simulink model "NPC_inverter_TS_203864"  (R2023b)
settings: Solver=ode4  StartTime=0.0  StopTime=Tsim  FixedStep=Ts  RelTol=1e-3
InitFcn:
  | run('param.m');
values from neighbouring files (symbols this model uses):
  f = 50    [param_nfE.m]
  mmax = 1    [param_nfE.m]
  mmin = -1    [param_nfE.m]
  TA = Tc    (= 0.000125)    [param_nfE.m]
  Tc = 1/fc    (= 0.000125)    [param_nfE.m]
  Umax = Ud/2    (= 350)    [param_nfE.m]
undefined symbols (not defined in the file or in its folder): plecs
libraries: simulink x12, plecslib x5
settings Model: Creator=timsp  LastModifiedBy=timsp

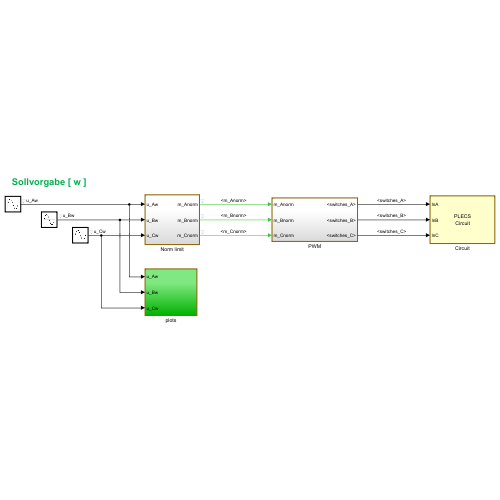
[thumbnail: Simulink's stored preview of the top-level diagram]
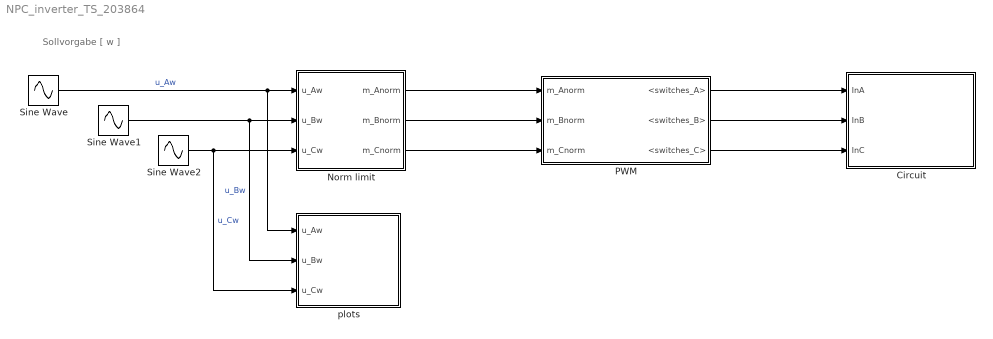
== system NPC_inverter_TS_203864 ==
  note: Sollvorgabe [ w ]
  Circuit : Subsystem  LoadFcn=plecs('sl', 200);  InitFcn=plecs('sl', 214);  StartFcn=plecs('sl', 208);  StopFcn=plecs('sl', 209);  mask(PlecsCircuit){PLECSData=<binary blob, 5248 chars, not shown>}
      mask prompts: PLECSData "PLECS Data (Do not delete or modify!)"
      mask init:
      | % PLACE CUSTOM INITIALIZATIONS ABOVE
      | % DO NOT REMOVE
      | plecs('sl', 215);
      | % DO NOT REMOVE
      settings: CopyFcn=plecs('sl', 203);  DeleteFcn=plecs('sl', 205);  UndoDeleteFcn=plecs('sl', 206);  PreSaveFcn=plecs('sl', 211);  PostSaveFcn=plecs('sl', 201);  NameChangeFcn=plecs('sl', 210);  DestroyFcn=plecs('sl', 207);  PreCopyFcn=plecs('sl', 216);  OpenFcn=plecs('sl', 202);  ErrorFcn=plerrorfcn
      mask Help: eval('plecs(''help'', ''qthelp:///creatingacircuit.html'')')
      mask Display: disp('PLECS\nCircuit')
  Norm limit : Subsystem
  PWM : Subsystem
  Sine Wave : Sin  Amplitude=Umax  Frequency=2*pi*f  Phase=pi/2  SampleTime=0
  Sine Wave1 : Sin  Amplitude=Umax  Frequency=2*pi*f  Phase=-2*pi/3+pi/2  SampleTime=0
  Sine Wave2 : Sin  Amplitude=Umax  Frequency=2*pi*f  Phase=-4*pi/3+pi/2  SampleTime=0
  plots : Subsystem
  wires:
  PWM/1(<switches_A>) -> Circuit/1(InA)
  PWM/2(<switches_B>) -> Circuit/2(InB)
  PWM/3(<switches_C>) -> Circuit/3(InC)
  Norm limit/1(m_Anorm) -> PWM/1(m_Anorm)
  Norm limit/2(m_Bnorm) -> PWM/2(m_Bnorm)
  Norm limit/3(m_Cnorm) -> PWM/3(m_Cnorm)
  Sine Wave/1 -> plots/1(u_Aw), Norm limit/1(u_Aw)  "u_Aw"
  Sine Wave1/1 -> plots/2(u_Bw), Norm limit/2(u_Bw)  "u_Bw"
  Sine Wave2/1 -> plots/3(u_Cw), Norm limit/3(u_Cw)  "u_Cw"

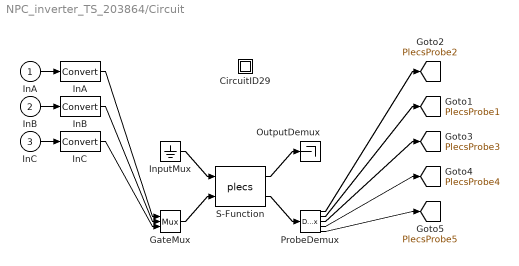
== system NPC_inverter_TS_203864/Circuit ==
  InA : Inport  PortDimensions=4
  InB : Inport  Port=2  PortDimensions=4
  InC : Inport  Port=3  PortDimensions=4
  " CircuitID29 " : Subsystem
  " GateMux " : Mux  Inputs=[ 4 4 4 ]
  " InA " : DataTypeConversion
  " InB " : DataTypeConversion
  " InC " : DataTypeConversion
  " InputMux " : Ground
  " OutputDemux " : Terminator
  " ProbeDemux " : Demux  Outputs=[ 3 3 3 1 3 ]
  " S-Function " : S-Function  FunctionName=plecs  SFunctionDeploymentMode=off  EnableBusSupport=off
  tag scope: PlecsProbe1=global, PlecsProbe2=global, PlecsProbe3=global, PlecsProbe4=global, PlecsProbe5=global
  wires:
  " InputMux "/1 -> " S-Function "/1
  " GateMux "/1 -> " S-Function "/2
  " S-Function "/1 -> " OutputDemux "/1
  " S-Function "/2 -> " ProbeDemux "/1
  InA/1 -> " InA "/1
  " InA "/1 -> " GateMux "/1
  InB/1 -> " InB "/1
  " InB "/1 -> " GateMux "/2
  InC/1 -> " InC "/1
  " InC "/1 -> " GateMux "/3
  " ProbeDemux "/1 -> [PlecsProbe2]
  " ProbeDemux "/2 -> [PlecsProbe1]
  " ProbeDemux "/3 -> [PlecsProbe3]
  " ProbeDemux "/4 -> [PlecsProbe4]
  " ProbeDemux "/5 -> [PlecsProbe5]

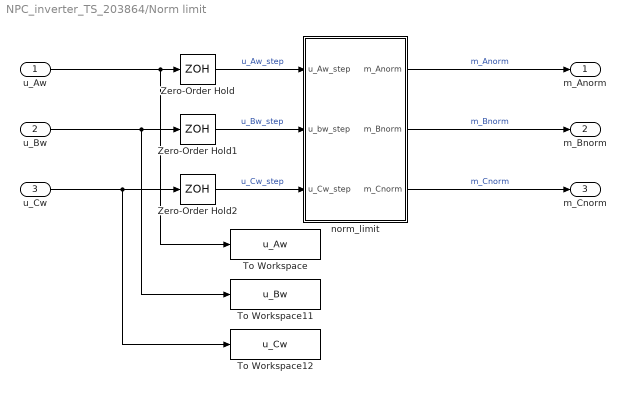
== system NPC_inverter_TS_203864/Norm limit ==
  u_Aw : Inport
  u_Bw : Inport  Port=2
  u_Cw : Inport  Port=3
  To Workspace : ToWorkspace  VariableName=u_Aw  SampleTime=-1
      settings: Save2DSignal=2-D array (concatenate along first dimension)
  To Workspace11 : ToWorkspace  VariableName=u_Bw  SampleTime=-1
      settings: Save2DSignal=2-D array (concatenate along first dimension)
  To Workspace12 : ToWorkspace  VariableName=u_Cw  SampleTime=-1
      settings: Save2DSignal=2-D array (concatenate along first dimension)
  Zero-Order Hold : ZeroOrderHold  SampleTime=TA
  Zero-Order Hold1 : ZeroOrderHold  SampleTime=TA
  Zero-Order Hold2 : ZeroOrderHold  SampleTime=TA
  norm_limit : Subsystem
  m_Anorm : Outport
  m_Bnorm : Outport  Port=2
  m_Cnorm : Outport  Port=3
  wires:
  u_Cw/1 -> To Workspace12/1, Zero-Order Hold2/1
  u_Bw/1 -> To Workspace11/1, Zero-Order Hold1/1
  norm_limit/3(m_Cnorm) -> m_Cnorm/1  "m_Cnorm"
  Zero-Order Hold1/1 -> norm_limit/2(u_bw_step)  "u_Bw_step"
  norm_limit/2(m_Bnorm) -> m_Bnorm/1  "m_Bnorm"
  Zero-Order Hold/1 -> norm_limit/1(u_Aw_step)  "u_Aw_step"
  Zero-Order Hold2/1 -> norm_limit/3(u_Cw_step)  "u_Cw_step"
  norm_limit/1(m_Anorm) -> m_Anorm/1  "m_Anorm"
  u_Aw/1 -> To Workspace/1, Zero-Order Hold/1

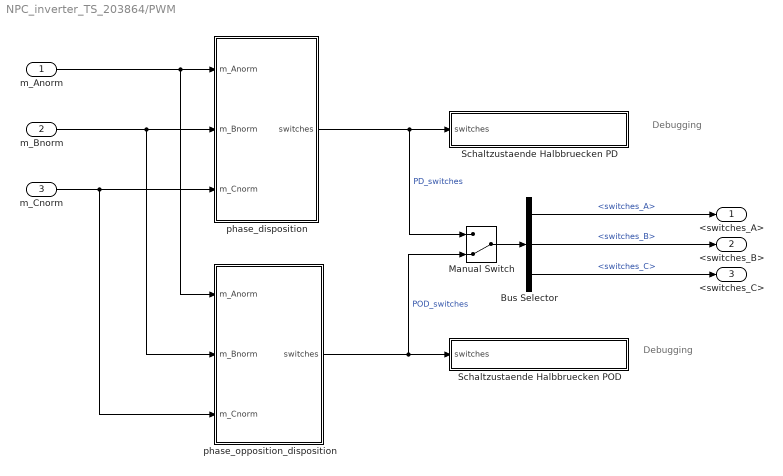
== system NPC_inverter_TS_203864/PWM ==
  note: Debugging
  note: Debugging
  m_Anorm : Inport
  m_Bnorm : Inport  Port=2
  m_Cnorm : Inport  Port=3
  Bus Selector : BusSelector  OutputSignals=switches_A,switches_B,switches_C
  Manual Switch : ManualSwitch  CurrentSetting=0
  Schaltzustaende Halbbruecken PD : Subsystem
  Schaltzustaende Halbbruecken POD : Subsystem
  phase_disposition : Subsystem  TreatAsAtomicUnit=on
  phase_opposition_disposition : Subsystem  TreatAsAtomicUnit=on
  <switches_A> : Outport
  <switches_B> : Outport  Port=2
  <switches_C> : Outport  Port=3
  wires:
  m_Bnorm/1 -> phase_disposition/2(m_Bnorm), phase_opposition_disposition/2(m_Bnorm)
  phase_disposition/1(switches) -> Schaltzustaende Halbbruecken PD/1(switches), Manual Switch/1  "PD_switches"
  phase_opposition_disposition/1(switches) -> Manual Switch/2, Schaltzustaende Halbbruecken POD/1(switches)  "POD_switches"
  Bus Selector/3 -> <switches_C>/1  "<switches_C>"
  m_Cnorm/1 -> phase_opposition_disposition/3(m_Cnorm), phase_disposition/3(m_Cnorm)
  m_Anorm/1 -> phase_opposition_disposition/1(m_Anorm), phase_disposition/1(m_Anorm)
  Bus Selector/1 -> <switches_A>/1  "<switches_A>"
  Manual Switch/1 -> Bus Selector/1
  Bus Selector/2 -> <switches_B>/1  "<switches_B>"

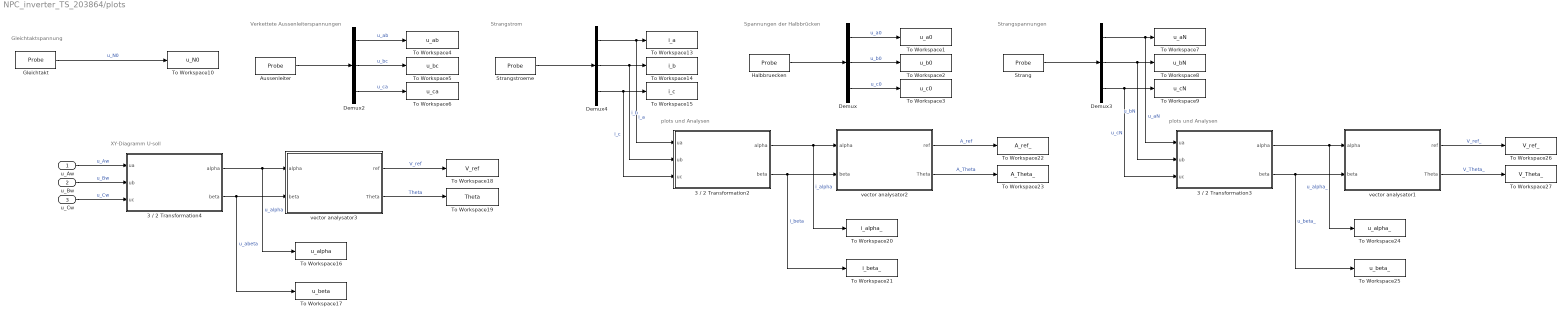
== system NPC_inverter_TS_203864/plots ==
  note: Gleichtaktspannung
  note: Spannungen der Halbbrücken
  note: Verkettete Aussenleiterspannungen
  note: Strangspannungen
  note: Strangstrom
  note: plots und Analysen
  note: plots und Analysen
  note: XY-Diagramm U-soll
  u_Aw : Inport
  u_Bw : Inport  Port=2
  u_Cw : Inport  Port=3
  3 / 2 Transformation2 : MATLAB Function  TreatAsAtomicUnit=on
  3 / 2 Transformation3 : MATLAB Function  TreatAsAtomicUnit=on
  3 / 2 Transformation4 : MATLAB Function  TreatAsAtomicUnit=on
  Aussenleiter : plecslib/Probe  tagno=1
      settings: SourceProductName=PLECS
  Demux{,2..4} (4 alike) : Demux  Outputs=3
  Gleichtakt : plecslib/Probe  tagno=4
      settings: SourceProductName=PLECS
  Halbbruecken : plecslib/Probe  tagno=2
      settings: SourceProductName=PLECS
  Strang : plecslib/Probe  tagno=3
      settings: SourceProductName=PLECS
  Strangstroeme : plecslib/Probe  tagno=5
      settings: SourceProductName=PLECS
  To Workspace1 : ToWorkspace  VariableName=u_a0  SampleTime=-1
  To Workspace10 : ToWorkspace  VariableName=u_N0  SampleTime=-1
  To Workspace13 : ToWorkspace  VariableName=i_a  SampleTime=-1
  To Workspace14 : ToWorkspace  VariableName=i_b  SampleTime=-1
  To Workspace15 : ToWorkspace  VariableName=i_c  SampleTime=-1
  To Workspace16 : ToWorkspace  VariableName=u_alpha  SampleTime=-1
  To Workspace17 : ToWorkspace  VariableName=u_beta  SampleTime=-1
  To Workspace18 : ToWorkspace  VariableName=V_ref  SampleTime=-1
  To Workspace19 : ToWorkspace  VariableName=Theta  SampleTime=-1
  To Workspace2 : ToWorkspace  VariableName=u_b0  SampleTime=-1
  To Workspace20 : ToWorkspace  VariableName=i_alpha_  SampleTime=-1
  To Workspace21 : ToWorkspace  VariableName=i_beta_  SampleTime=-1
  To Workspace22 : ToWorkspace  VariableName=A_ref_  SampleTime=-1
  To Workspace23 : ToWorkspace  VariableName=A_Theta_  SampleTime=-1
  To Workspace24 : ToWorkspace  VariableName=u_alpha_  SampleTime=-1
  To Workspace25 : ToWorkspace  VariableName=u_beta_  SampleTime=-1
  To Workspace26 : ToWorkspace  VariableName=V_ref_  SampleTime=-1
  To Workspace27 : ToWorkspace  VariableName=V_Theta_  SampleTime=-1
  To Workspace3 : ToWorkspace  VariableName=u_c0  SampleTime=-1
  To Workspace4 : ToWorkspace  VariableName=u_ab  SampleTime=-1
  To Workspace5 : ToWorkspace  VariableName=u_bc  SampleTime=-1
  To Workspace6 : ToWorkspace  VariableName=u_ca  SampleTime=-1
  To Workspace7 : ToWorkspace  VariableName=u_aN  SampleTime=-1
  To Workspace8 : ToWorkspace  VariableName=u_bN  SampleTime=-1
  To Workspace9 : ToWorkspace  VariableName=u_cN  SampleTime=-1
  vector analysator1 : MATLAB Function  TreatAsAtomicUnit=on
  vector analysator2 : MATLAB Function  TreatAsAtomicUnit=on
  vector analysator3 : MATLAB Function  TreatAsAtomicUnit=on
  wires:
  Demux3/3 -> 3 / 2 Transformation3/3(uc), To Workspace9/1  "u_cN"
  Demux2/1 -> To Workspace4/1  "u_ab"
  Demux2/2 -> To Workspace5/1  "u_bc"
  Aussenleiter/1 -> Demux2/1
  vector analysator1/2(Theta) -> To Workspace27/1  "V_Theta_"
  Demux4/2 -> 3 / 2 Transformation2/2(ub), To Workspace14/1  "i_b"
  Demux3/2 -> 3 / 2 Transformation3/2(ub), To Workspace8/1  "u_bN"
  3 / 2 Transformation3/2(beta) -> vector analysator1/2(beta), To Workspace25/1  "u_beta_"
  Strangstroeme/1 -> Demux4/1
  Demux/1 -> To Workspace1/1  "u_a0"
  Gleichtakt/1 -> To Workspace10/1  "u_N0"
  Demux/2 -> To Workspace2/1  "u_b0"
  Demux4/3 -> 3 / 2 Transformation2/3(uc), To Workspace15/1  "i_c"
  Demux2/3 -> To Workspace6/1  "u_ca"
  3 / 2 Transformation3/1(alpha) -> vector analysator1/1(alpha), To Workspace24/1  "u_alpha_"
  3 / 2 Transformation2/2(beta) -> vector analysator2/2(beta), To Workspace21/1  "i_beta"
  vector analysator2/2(Theta) -> To Workspace23/1  "A_Theta"
  Demux4/1 -> 3 / 2 Transformation2/1(ua), To Workspace13/1  "i_a"
  vector analysator2/1(ref) -> To Workspace22/1  "A_ref"
  3 / 2 Transformation2/1(alpha) -> vector analysator2/1(alpha), To Workspace20/1  "i_alpha"
  vector analysator1/1(ref) -> To Workspace26/1  "V_ref_"
  Strang/1 -> Demux3/1
  Demux3/1 -> 3 / 2 Transformation3/1(ua), To Workspace7/1  "u_aN"
  Halbbruecken/1 -> Demux/1
  Demux/3 -> To Workspace3/1  "u_c0"
  vector analysator3/2(Theta) -> To Workspace19/1  "Theta"
  u_Cw/1 -> 3 / 2 Transformation4/3(uc)  "u_Cw"
  3 / 2 Transformation4/2(beta) -> vector analysator3/2(beta), To Workspace17/1  "u_abeta"
  vector analysator3/1(ref) -> To Workspace18/1  "V_ref"
  3 / 2 Transformation4/1(alpha) -> vector analysator3/1(alpha), To Workspace16/1  "u_alpha"
  u_Bw/1 -> 3 / 2 Transformation4/2(ub)  "u_Bw"
  u_Aw/1 -> 3 / 2 Transformation4/1(ua)  "u_Aw"

== system NPC_inverter_TS_203864/Circuit/ CircuitID29  ==

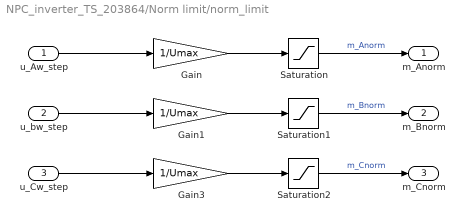
== system NPC_inverter_TS_203864/Norm limit/norm_limit ==
  u_Aw_step : Inport
  u_bw_step : Inport  Port=2
  u_Cw_step : Inport  Port=3
  Gain : Gain  Gain=1/Umax
  Gain1 : Gain  Gain=1/Umax
  Gain3 : Gain  Gain=1/Umax
  Saturation : Saturate  UpperLimit=mmax  LowerLimit=mmin
  Saturation1 : Saturate  UpperLimit=mmax  LowerLimit=mmin
  Saturation2 : Saturate  UpperLimit=mmax  LowerLimit=mmin
  m_Anorm : Outport
  m_Bnorm : Outport  Port=2
  m_Cnorm : Outport  Port=3
  wires:
  Gain/1 -> Saturation/1
  Gain3/1 -> Saturation2/1
  u_Cw_step/1 -> Gain3/1
  Gain1/1 -> Saturation1/1
  u_bw_step/1 -> Gain1/1
  u_Aw_step/1 -> Gain/1
  Saturation/1 -> m_Anorm/1  "m_Anorm"
  Saturation1/1 -> m_Bnorm/1  "m_Bnorm"
  Saturation2/1 -> m_Cnorm/1  "m_Cnorm"

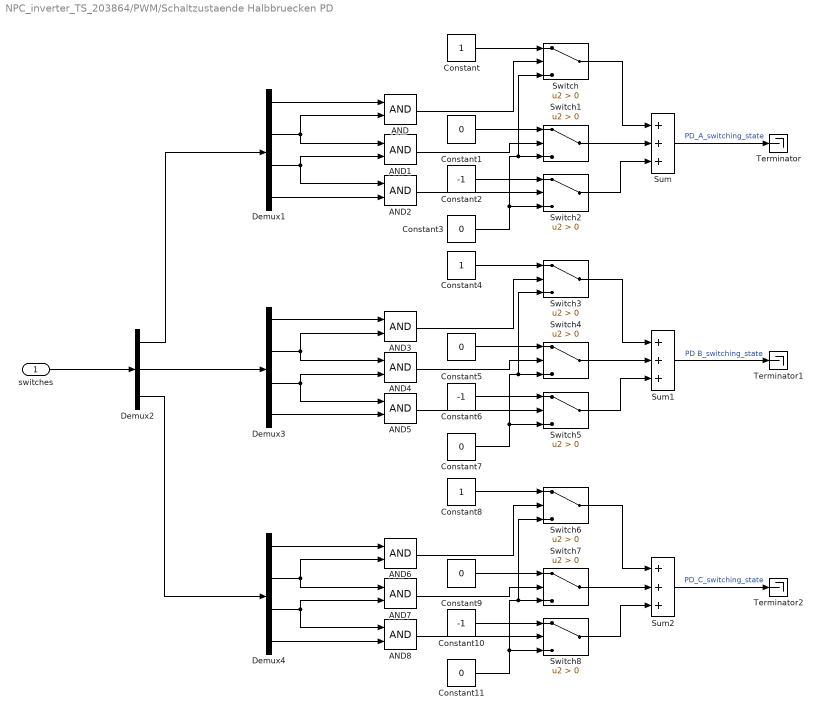
== system NPC_inverter_TS_203864/PWM/Schaltzustaende Halbbruecken PD ==
  switches : Inport
  AND{,1..8} (9 alike) : Logic  AllPortsSameDT=off  OutDataTypeStr=boolean
  Constant : Constant
  Constant{1,3,5,7,9,11} (6 alike) : Constant  Value=0
  Constant10 : Constant  Value=-1
  Constant2 : Constant  Value=-1
  Constant4 : Constant
  Constant6 : Constant  Value=-1
  Constant8 : Constant
  Demux1 : Demux
  Demux2 : Demux  Outputs=3
  Demux3 : Demux
  Demux4 : Demux
  Sum : Sum  Inputs=+++
  Sum1 : Sum  Inputs=+++
  Sum2 : Sum  Inputs=+++
  Switch{,1..8} (9 alike) : Switch  Criteria=u2 > Threshold  SaturateOnIntegerOverflow=off  InputSameDT=off
  Terminator : Terminator
  Terminator1 : Terminator
  Terminator2 : Terminator
  wires:
  Sum2/1 -> Terminator2/1  "PD_C_switching_state"
  Switch8/1 -> Sum2/3
  Switch7/1 -> Sum2/2
  Switch6/1 -> Sum2/1
  Constant11/1 -> Switch8/3, Switch7/3, Switch6/3
  Constant10/1 -> Switch8/1
  AND8/1 -> Switch8/2
  Constant9/1 -> Switch7/1
  AND7/1 -> Switch7/2
  Constant8/1 -> Switch6/1
  AND6/1 -> Switch6/2
  Demux4/4 -> AND8/2
  Demux4/3 -> AND7/2, AND8/1
  Demux4/2 -> AND6/2, AND7/1
  Demux4/1 -> AND6/1
  Demux3/1 -> AND3/1
  Demux3/2 -> AND4/1, AND3/2
  Demux3/3 -> AND5/1, AND4/2
  Demux3/4 -> AND5/2
  AND3/1 -> Switch3/2
  Constant4/1 -> Switch3/1
  AND4/1 -> Switch4/2
  Constant5/1 -> Switch4/1
  AND5/1 -> Switch5/2
  Constant6/1 -> Switch5/1
  Constant7/1 -> Switch3/3, Switch4/3, Switch5/3
  Switch3/1 -> Sum1/1
  Switch4/1 -> Sum1/2
  Switch5/1 -> Sum1/3
  Sum1/1 -> Terminator1/1  "PD B_switching_state"
  Sum/1 -> Terminator/1  "PD_A_switching_state"
  Switch2/1 -> Sum/3
  Switch1/1 -> Sum/2
  Switch/1 -> Sum/1
  Constant3/1 -> Switch2/3, Switch1/3, Switch/3
  Constant2/1 -> Switch2/1
  AND2/1 -> Switch2/2
  Constant1/1 -> Switch1/1
  AND1/1 -> Switch1/2
  Constant/1 -> Switch/1
  AND/1 -> Switch/2
  Demux2/2 -> Demux3/1
  Demux1/4 -> AND2/2
  Demux1/3 -> AND1/2, AND2/1
  Demux1/2 -> AND/2, AND1/1
  Demux1/1 -> AND/1
  Demux2/3 -> Demux4/1
  Demux2/1 -> Demux1/1
  switches/1 -> Demux2/1

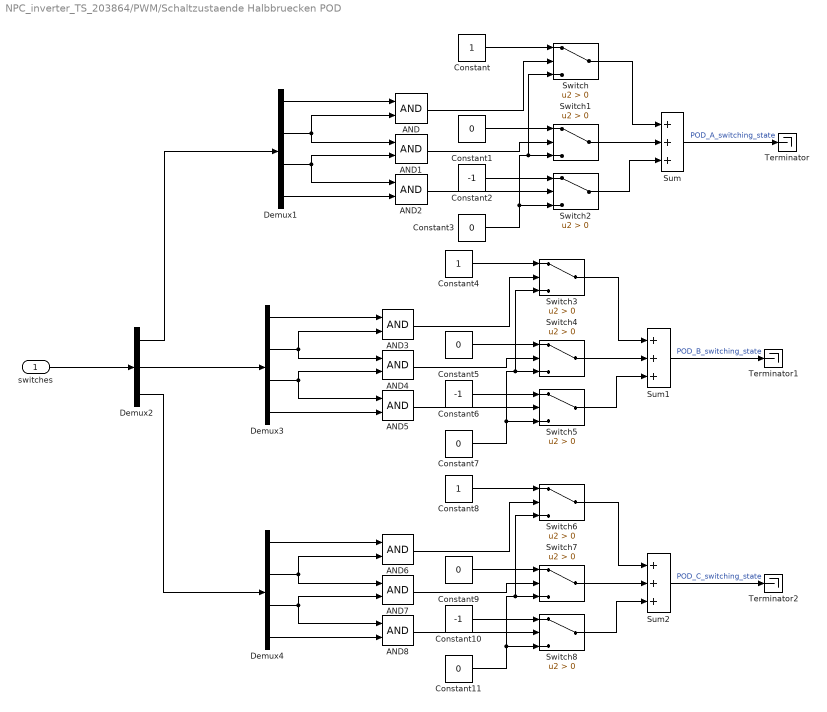
== system NPC_inverter_TS_203864/PWM/Schaltzustaende Halbbruecken POD ==
  switches : Inport
  AND{,1..8} (9 alike) : Logic  AllPortsSameDT=off  OutDataTypeStr=boolean
  Constant : Constant
  Constant{1,3,5,7,9,11} (6 alike) : Constant  Value=0
  Constant10 : Constant  Value=-1
  Constant2 : Constant  Value=-1
  Constant4 : Constant
  Constant6 : Constant  Value=-1
  Constant8 : Constant
  Demux1 : Demux
  Demux2 : Demux  Outputs=3
  Demux3 : Demux
  Demux4 : Demux
  Sum : Sum  Inputs=+++
  Sum1 : Sum  Inputs=+++
  Sum2 : Sum  Inputs=+++
  Switch{,1..8} (9 alike) : Switch  Criteria=u2 > Threshold  SaturateOnIntegerOverflow=off  InputSameDT=off
  Terminator : Terminator
  Terminator1 : Terminator
  Terminator2 : Terminator
  wires:
  switches/1 -> Demux2/1
  Demux2/1 -> Demux1/1
  Demux2/3 -> Demux4/1
  Demux1/1 -> AND/1
  Demux1/2 -> AND1/1, AND/2
  Demux1/3 -> AND2/1, AND1/2
  Demux1/4 -> AND2/2
  Demux2/2 -> Demux3/1
  AND/1 -> Switch/2
  Constant/1 -> Switch/1
  AND1/1 -> Switch1/2
  Constant1/1 -> Switch1/1
  AND2/1 -> Switch2/2
  Constant2/1 -> Switch2/1
  Constant3/1 -> Switch/3, Switch1/3, Switch2/3
  Switch/1 -> Sum/1
  Switch1/1 -> Sum/2
  Switch2/1 -> Sum/3
  Sum/1 -> Terminator/1  "POD_A_switching_state"
  Sum1/1 -> Terminator1/1  "POD_B_switching_state"
  Switch5/1 -> Sum1/3
  Switch4/1 -> Sum1/2
  Switch3/1 -> Sum1/1
  Constant7/1 -> Switch5/3, Switch4/3, Switch3/3
  Constant6/1 -> Switch5/1
  AND5/1 -> Switch5/2
  Constant5/1 -> Switch4/1
  AND4/1 -> Switch4/2
  Constant4/1 -> Switch3/1
  AND3/1 -> Switch3/2
  Demux3/4 -> AND5/2
  Demux3/3 -> AND4/2, AND5/1
  Demux3/2 -> AND3/2, AND4/1
  Demux3/1 -> AND3/1
  Demux4/1 -> AND6/1
  Demux4/2 -> AND7/1, AND6/2
  Demux4/3 -> AND8/1, AND7/2
  Demux4/4 -> AND8/2
  AND6/1 -> Switch6/2
  Constant8/1 -> Switch6/1
  AND7/1 -> Switch7/2
  Constant9/1 -> Switch7/1
  AND8/1 -> Switch8/2
  Constant10/1 -> Switch8/1
  Constant11/1 -> Switch6/3, Switch7/3, Switch8/3
  Switch6/1 -> Sum2/1
  Switch7/1 -> Sum2/2
  Switch8/1 -> Sum2/3
  Sum2/1 -> Terminator2/1  "POD_C_switching_state"

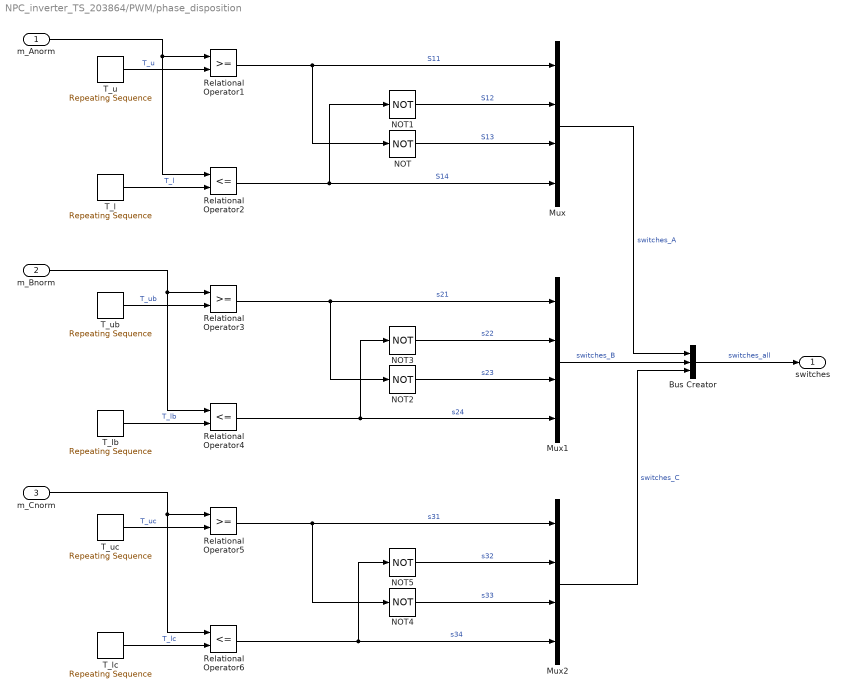
== system NPC_inverter_TS_203864/PWM/phase_disposition ==
  m_Anorm : Inport
  m_Bnorm : Inport  Port=2
  m_Cnorm : Inport  Port=3
  Bus Creator : BusCreator  Inputs=3
  Mux : Mux
  Mux1 : Mux
  Mux2 : Mux
  NOT{,1..5} (6 alike) : Logic  Operator=NOT  AllPortsSameDT=off  OutDataTypeStr=boolean
  Relational Operator1 : RelationalOperator  OutDataTypeStr=boolean  RndMeth=Simplest  InputSameDT=off
  Relational Operator2 : RelationalOperator  Operator=<=  OutDataTypeStr=boolean  RndMeth=Simplest  InputSameDT=off
  Relational Operator3 : RelationalOperator  OutDataTypeStr=boolean  RndMeth=Simplest  InputSameDT=off
  Relational Operator4 : RelationalOperator  Operator=<=  OutDataTypeStr=boolean  RndMeth=Simplest  InputSameDT=off
  Relational Operator5 : RelationalOperator  OutDataTypeStr=boolean  RndMeth=Simplest  InputSameDT=off
  Relational Operator6 : RelationalOperator  Operator=<=  OutDataTypeStr=boolean  RndMeth=Simplest  InputSameDT=off
  T_l : simulink/Sources/Repeating Sequence  rep_seq_t=[0 Tc/2 Tc]  rep_seq_y=[-1 0 -1]
  T_lb : simulink/Sources/Repeating Sequence  rep_seq_t=[0 Tc/2 Tc]  rep_seq_y=[-1 0 -1]
  T_lc : simulink/Sources/Repeating Sequence  rep_seq_t=[0 Tc/2 Tc]  rep_seq_y=[-1 0 -1]
  T_u : simulink/Sources/Repeating Sequence  rep_seq_t=[0 Tc/2 Tc]  rep_seq_y=[0 1 0]
  T_ub : simulink/Sources/Repeating Sequence  rep_seq_t=[0 Tc/2 Tc]  rep_seq_y=[0 1 0]
  T_uc : simulink/Sources/Repeating Sequence  rep_seq_t=[0 Tc/2 Tc]  rep_seq_y=[0 1 0]
  switches : Outport
  wires:
  Bus Creator/1 -> switches/1  "switches_all"
  m_Anorm/1 -> Relational Operator2/1, Relational Operator1/1
  Relational Operator1/1 -> NOT/1, Mux/1  "S11"
  Relational Operator2/1 -> NOT1/1, Mux/4  "S14"
  T_l/1 -> Relational Operator2/2  "T_l"
  T_u/1 -> Relational Operator1/2  "T_u"
  NOT/1 -> Mux/3  "S13"
  NOT1/1 -> Mux/2  "S12"
  NOT2/1 -> Mux1/3  "s23"
  NOT3/1 -> Mux1/2  "s22"
  T_lb/1 -> Relational Operator4/2  "T_lb"
  Relational Operator3/1 -> NOT2/1, Mux1/1  "s21"
  Relational Operator4/1 -> Mux1/4, NOT3/1  "s24"
  T_ub/1 -> Relational Operator3/2  "T_ub"
  T_uc/1 -> Relational Operator5/2  "T_uc"
  Relational Operator6/1 -> Mux2/4, NOT5/1  "s34"
  T_lc/1 -> Relational Operator6/2  "T_lc"
  NOT4/1 -> Mux2/3  "s33"
  Relational Operator5/1 -> NOT4/1, Mux2/1  "s31"
  NOT5/1 -> Mux2/2  "s32"
  Mux/1 -> Bus Creator/1  "switches_A"
  Mux1/1 -> Bus Creator/2  "switches_B"
  Mux2/1 -> Bus Creator/3  "switches_C"
  m_Cnorm/1 -> Relational Operator6/1, Relational Operator5/1
  m_Bnorm/1 -> Relational Operator4/1, Relational Operator3/1

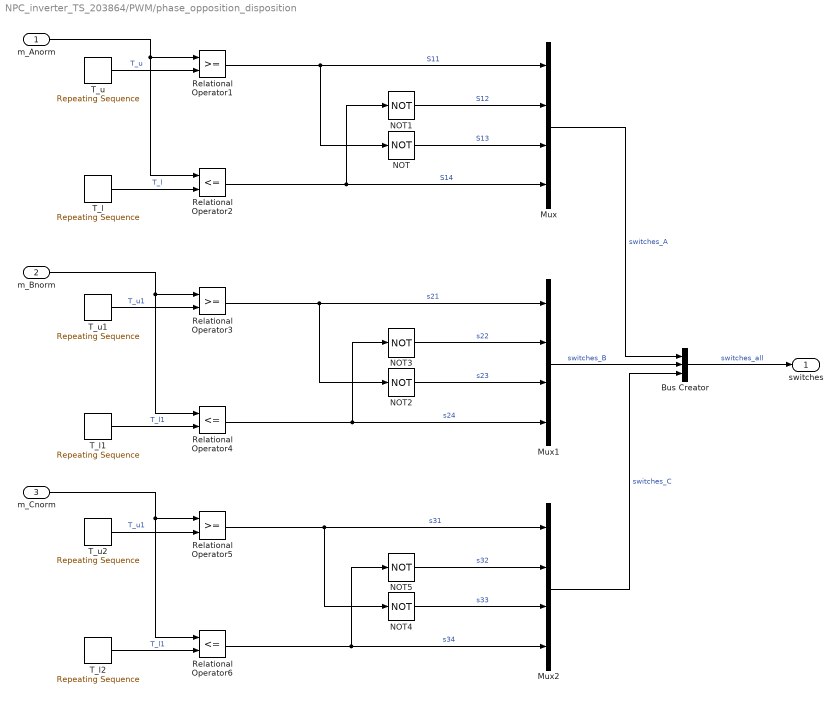
== system NPC_inverter_TS_203864/PWM/phase_opposition_disposition ==
  m_Anorm : Inport
  m_Bnorm : Inport  Port=2
  m_Cnorm : Inport  Port=3
  Bus Creator : BusCreator  Inputs=3
  Mux : Mux
  Mux1 : Mux
  Mux2 : Mux
  NOT{,1..5} (6 alike) : Logic  Operator=NOT  AllPortsSameDT=off  OutDataTypeStr=boolean
  Relational Operator1 : RelationalOperator  OutDataTypeStr=boolean  RndMeth=Simplest  InputSameDT=off
  Relational Operator2 : RelationalOperator  Operator=<=  OutDataTypeStr=boolean  RndMeth=Simplest  InputSameDT=off
  Relational Operator3 : RelationalOperator  OutDataTypeStr=boolean  RndMeth=Simplest  InputSameDT=off
  Relational Operator4 : RelationalOperator  Operator=<=  OutDataTypeStr=boolean  RndMeth=Simplest  InputSameDT=off
  Relational Operator5 : RelationalOperator  OutDataTypeStr=boolean  RndMeth=Simplest  InputSameDT=off
  Relational Operator6 : RelationalOperator  Operator=<=  OutDataTypeStr=boolean  RndMeth=Simplest  InputSameDT=off
  T_l : simulink/Sources/Repeating Sequence  rep_seq_t=[0 Tc/2 Tc]  rep_seq_y=[ 0 -1 0]
  T_l1 : simulink/Sources/Repeating Sequence  rep_seq_t=[0 Tc/2 Tc]  rep_seq_y=[0 -1 0]
  T_l2 : simulink/Sources/Repeating Sequence  rep_seq_t=[0 Tc/2 Tc]  rep_seq_y=[0 -1 0]
  T_u : simulink/Sources/Repeating Sequence  rep_seq_t=[0 Tc/2 Tc]  rep_seq_y=[0 1 0]
  T_u1 : simulink/Sources/Repeating Sequence  rep_seq_t=[0 Tc/2 Tc]  rep_seq_y=[0 1 0]
  T_u2 : simulink/Sources/Repeating Sequence  rep_seq_t=[0 Tc/2 Tc]  rep_seq_y=[0 1 0]
  switches : Outport
  wires:
  Relational Operator6/1 -> NOT5/1, Mux2/4  "s34"
  Bus Creator/1 -> switches/1  "switches_all"
  Relational Operator3/1 -> NOT2/1, Mux1/1  "s21"
  m_Anorm/1 -> Relational Operator2/1, Relational Operator1/1
  T_u/1 -> Relational Operator1/2  "T_u"
  T_l/1 -> Relational Operator2/2  "T_l"
  NOT2/1 -> Mux1/3  "s23"
  Relational Operator1/1 -> Mux/1, NOT/1  "S11"
  Relational Operator2/1 -> Mux/4, NOT1/1  "S14"
  NOT1/1 -> Mux/2  "S12"
  Mux2/1 -> Bus Creator/3  "switches_C"
  NOT3/1 -> Mux1/2  "s22"
  NOT4/1 -> Mux2/3  "s33"
  m_Bnorm/1 -> Relational Operator4/1, Relational Operator3/1
  NOT5/1 -> Mux2/2  "s32"
  T_u2/1 -> Relational Operator5/2  "T_u1"
  Mux1/1 -> Bus Creator/2  "switches_B"
  NOT/1 -> Mux/3  "S13"
  Relational Operator4/1 -> NOT3/1, Mux1/4  "s24"
  Relational Operator5/1 -> Mux2/1, NOT4/1  "s31"
  T_u1/1 -> Relational Operator3/2  "T_u1"
  Mux/1 -> Bus Creator/1  "switches_A"
  T_l1/1 -> Relational Operator4/2  "T_l1"
  m_Cnorm/1 -> Relational Operator6/1, Relational Operator5/1
  T_l2/1 -> Relational Operator6/2  "T_l1"

== matlab function NPC_inverter_TS_203864/plots/vector analysator3 ==
  data: alpha input; ref output; Theta output; beta input
function [ref, Theta]= fcn(alpha, beta)
% ### input vector ###
% u1 = alpha (real part or space vector)
% u2 = beta (imaginary part of space vector)

% ### output vector ###
% y1 = ref (absolute value)
% y2 = Theta (angle)

% ### calculation ####
    ref = sqrt(alpha^2+beta^2);

    Theta = atan2(beta, alpha); % damit Theta [0, 2pi]

end

== matlab function NPC_inverter_TS_203864/plots/vector analysator1 ==
  data: alpha input; ref output; Theta output; beta input
function [ref, Theta]= fcn(alpha, beta)
% ### input vector ###
% u1 = alpha (real part or space vector)
% u2 = beta (imaginary part of space vector)

% ### output vector ###
% y1 = ref (absolute value)
% y2 = Theta (angle)

% ### calculation ####
    ref = sqrt(alpha^2+beta^2);

    Theta = atan2(beta, alpha); % damit Theta [0, 2pi]

end

== matlab function NPC_inverter_TS_203864/plots/3 // 2 Transformation2 ==
  data: ua input; alpha output; ub input; uc input; beta output
function [alpha, beta] = fcn(ua, ub, uc)
% ### input vector ###
% u1 = ua
% u2 = ub
% u3 = uc

% ### output vector ###
% y1 = alpha
% y2 = beta
% y3 = u_0

% ### calculation ###
    T = 2/3.*   [1 -1/2 -1/2;...
                0 sqrt(3)/2 -sqrt(3)/2;...
                1/2 1/2 1/2];
    
    y = T * [ua; ub; uc];   
    
% ### return ###
    alpha = y(1);
    beta = y(2);
    %u_0 = y(3);
end

== matlab function NPC_inverter_TS_203864/plots/3 // 2 Transformation4 ==
  data: ua input; alpha output; ub input; uc input; beta output
function [alpha, beta] = fcn(ua, ub, uc)
% ### input vector ###
% u1 = ua
% u2 = ub
% u3 = uc

% ### output vector ###
% y1 = alpha
% y2 = beta
% y3 = u_0

% ### calculation ###
    T = 2/3.*   [1 -1/2 -1/2;...
                0 sqrt(3)/2 -sqrt(3)/2;...
                1/2 1/2 1/2];
    
    y = T * [ua; ub; uc];   
    
% ### return ###
    alpha = y(1);
    beta = y(2);
    %u_0 = y(3);
end

== matlab function NPC_inverter_TS_203864/plots/vector analysator2 ==
  data: alpha input; ref output; Theta output; beta input
function [ref, Theta]= fcn(alpha, beta)
% ### input vector ###
% u1 = alpha (real part or space vector)
% u2 = beta (imaginary part of space vector)

% ### output vector ###
% y1 = ref (absolute value)
% y2 = Theta (angle)

% ### calculation ####
    ref = sqrt(alpha^2+beta^2);

    Theta = atan2(beta, alpha); % damit Theta [0, 2pi]

end

== matlab function NPC_inverter_TS_203864/plots/3 // 2 Transformation3 ==
  data: ua input; alpha output; ub input; uc input; beta output
function [alpha, beta] = fcn(ua, ub, uc)
% ### input vector ###
% u1 = ua
% u2 = ub
% u3 = uc

% ### output vector ###
% y1 = alpha
% y2 = beta
% y3 = u_0

% ### calculation ###
    T = 2/3.*   [1 -1/2 -1/2;...
                0 sqrt(3)/2 -sqrt(3)/2;...
                1/2 1/2 1/2];
    
    y = T * [ua; ub; uc];   
    
% ### return ###
    alpha = y(1);
    beta = y(2);
    %u_0 = y(3);
end
